simulink library "adcs_fsw_main"  (R2016b)
settings: Solver=ode45  StartTime=0.0  StopTime=10.0  RelTol=1e-3  EnableMultiTasking=on
undefined symbols (not defined in the file): MT_dv, RW_rpm
libraries: CAN_lib x1, MSP_BDOT_lib x1, MSP_FSW_lib x1, MSP_MT_lib x1, bus_stubs_template x1, sensor_processing x1
settings Model: Creator=bbarz_000  LastModifiedBy=Taylor
settings DataIOCC: LimitDataPoints=on
settings OptimizationCC: LifeSpan=inf
settings DebuggingCC: AllowSymbolicDim=off  SFUnexpectedBacktrackingDiag=warning  SFNoUnconditionalDefaultTransitionDiag=warning  SFExecutionAtInitializationDiag=none
settings GRTTargetCC: TargetLangStandard=C89/C90 (ANSI)  GeneratePreprocessorConditionals=Disable all
settings ConfigComp: CovMetricSettings=dw  CovHtmlReporting=on  CovSaveCumulativeToWorkspaceVar=on  CovSaveSingleToWorkspaceVar=on  CovExternalEMLEnable=off

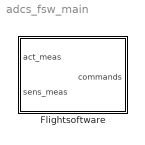
== system adcs_fsw_main ==
  Flightsoftware : Subsystem

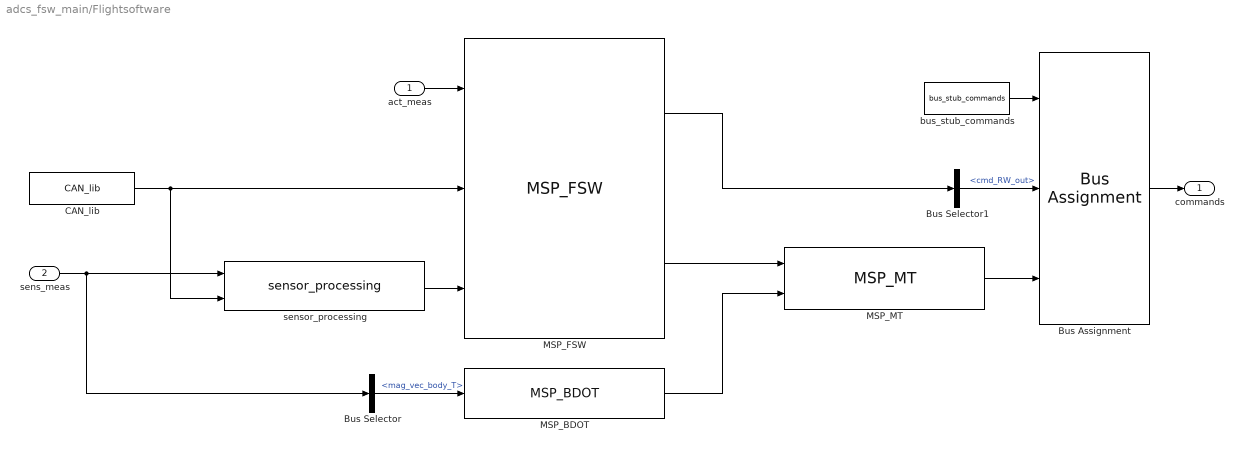
== system adcs_fsw_main/Flightsoftware ==
  act_meas : Inport  OutDataTypeStr=Bus: act_meas
  sens_meas : Inport  Port=2  OutDataTypeStr=Bus: sens_meas
  Bus Assignment : BusAssignment  AssignedSignals=RW_rpm,MT_dv
  Bus Selector : BusSelector  OutputSignals=mag_vec_body_T
  Bus Selector1 : BusSelector  OutputSignals=cmd_RW_out
  CAN_lib : CAN_lib/CAN_lib
  MSP_BDOT : MSP_BDOT_lib/MSP_BDOT
  MSP_FSW : MSP_FSW_lib/MSP_FSW
  MSP_MT : MSP_MT_lib/MSP_MT
  bus_stub_commands : bus_stubs_template/bus_stub_commands
  sensor_processing : sensor_processing/sensor_processing
  commands : Outport
  wires:
  Bus Assignment/1 -> commands/1
  bus_stub_commands/1 -> Bus Assignment/1
  sens_meas/1 -> Bus Selector/1, sensor_processing/1
  Bus Selector/1 -> MSP_BDOT/1  "<mag_vec_body_T>"
  MSP_MT/1 -> Bus Assignment/3
  MSP_BDOT/1 -> MSP_MT/2
  act_meas/1 -> MSP_FSW/1
  CAN_lib/1 -> sensor_processing/2, MSP_FSW/2
  MSP_FSW/1 -> Bus Selector1/1
  sensor_processing/1 -> MSP_FSW/3
  Bus Selector1/1 -> Bus Assignment/2  "<cmd_RW_out>"
  MSP_FSW/2 -> MSP_MT/1
